simulink model "SPGF_FSK_0000_R2022b"  (R2022b)
settings: Solver=ode4  StartTime=0.0  StopTime=1.4  FixedStep=50e-6/50  RelTol=1e-3  EnableMultiTasking=on
undefined symbols (not defined in the file): D11, Delta
libraries: spsSeriesRLCBranchLib x1646, spsGroundLib x360, spsStairGeneratorLib x147, spsIdealSwitchLib x145, spsCurrentMeasurementLib x145, spsUniversalBridgeLib x76, spsThreePhaseSeriesRLCLoadLib x57, simulink x45, spsBistableLib x36, spsSequenceAnalyzerLib x31, spsThreePhaseParallelRLCLoadLib x20, spsThreePhaseTransformerTwoWindingsLib x20
(part 17 of 40)

== system SPGF_FSK_0000_R2022b/W12/concentrated ==
  Ccs/1 : spsSeriesRLCBranchLib/Series RLC Branch  LConnTagsString=__new0  RConnTagsString=__new0  BranchType=C  Resistance=190  Inductance=1e-3  SetiL0=off  InitialCurrent=0  Capacitance=-C_matrix(1,2)/2  Setx0=off  InitialVoltage=0  Measurements=None
  Ccs/2 : spsSeriesRLCBranchLib/Series RLC Branch  LConnTagsString=__new0  RConnTagsString=__new0  BranchType=C  Resistance=190  Inductance=1e-3  SetiL0=off  InitialCurrent=0  Capacitance=-C_matrix(1,2)/2  Setx0=off  InitialVoltage=0  Measurements=None
  Ccs2/1 : spsSeriesRLCBranchLib/Series RLC Branch  LConnTagsString=__new0  RConnTagsString=__new0  BranchType=C  Resistance=190  Inductance=1e-3  SetiL0=off  InitialCurrent=0  Capacitance=-C_matrix(3,4)/2  Setx0=off  InitialVoltage=0  Measurements=None
  Ccs2/2 : spsSeriesRLCBranchLib/Series RLC Branch  LConnTagsString=__new0  RConnTagsString=__new0  BranchType=C  Resistance=190  Inductance=1e-3  SetiL0=off  InitialCurrent=0  Capacitance=-C_matrix(3,4)/2  Setx0=off  InitialVoltage=0  Measurements=None
  Ccs2/3 : spsSeriesRLCBranchLib/Series RLC Branch  LConnTagsString=__new0  RConnTagsString=__new0  BranchType=R  Resistance=-Rg_matrix(3,4)*2  Inductance=1e-3  SetiL0=off  InitialCurrent=0  Capacitance=Rg_matrix(3,4)*2  Setx0=off  InitialVoltage=0  Measurements=None
  Ccs2/4 : spsSeriesRLCBranchLib/Series RLC Branch  LConnTagsString=__new0  RConnTagsString=__new0  BranchType=R  Resistance=-Rg_matrix(3,4)*2  Inductance=1e-3  SetiL0=off  InitialCurrent=0  Capacitance=Rg_matrix(3,4)*2  Setx0=off  InitialVoltage=0  Measurements=None
  Ccs3/1 : spsSeriesRLCBranchLib/Series RLC Branch  LConnTagsString=__new0  RConnTagsString=__new0  BranchType=C  Resistance=190  Inductance=1e-3  SetiL0=off  InitialCurrent=0  Capacitance=-C_matrix(5,6)/2  Setx0=off  InitialVoltage=0  Measurements=None
  Ccs3/2 : spsSeriesRLCBranchLib/Series RLC Branch  LConnTagsString=__new0  RConnTagsString=__new0  BranchType=C  Resistance=190  Inductance=1e-3  SetiL0=off  InitialCurrent=0  Capacitance=-C_matrix(5,6)/2  Setx0=off  InitialVoltage=0  Measurements=None
  Ccs3/3 : spsSeriesRLCBranchLib/Series RLC Branch  LConnTagsString=__new0  RConnTagsString=__new0  BranchType=R  Resistance=-Rg_matrix(5,6)*2  Inductance=1e-3  SetiL0=off  InitialCurrent=0  Capacitance=-C_matrix(5,6)/2  Setx0=off  InitialVoltage=0  Measurements=None
  Ccs3/4 : spsSeriesRLCBranchLib/Series RLC Branch  LConnTagsString=__new0  RConnTagsString=__new0  BranchType=R  Resistance=-Rg_matrix(5,6)*2  Inductance=1e-3  SetiL0=off  InitialCurrent=0  Capacitance=-C_matrix(5,6)/2  Setx0=off  InitialVoltage=0  Measurements=None
  Csg/2 : spsSeriesRLCBranchLib/Series RLC Branch  LConnTagsString=__new0  RConnTagsString=__new0  BranchType=C  Resistance=190  Inductance=1e-3  SetiL0=off  InitialCurrent=0  Capacitance=( C_matrix(1,2) + C_matrix(2,2) )/2  Setx0=off  InitialVoltage=0  Measurements=None
  Csg1/1 : spsSeriesRLCBranchLib/Series RLC Branch  LConnTagsString=__new0  RConnTagsString=__new0  BranchType=C  Resistance=190  Inductance=1e-3  SetiL0=off  InitialCurrent=0  Capacitance=( C_matrix(1,2) + C_matrix(2,2) )/2  Setx0=off  InitialVoltage=0  Measurements=None
  Csg2/1 : spsSeriesRLCBranchLib/Series RLC Branch  LConnTagsString=__new0  RConnTagsString=__new0  BranchType=C  Resistance=190  Inductance=1e-3  SetiL0=off  InitialCurrent=0  Capacitance=( C_matrix(3,4) + C_matrix(4,4) )/2  Setx0=off  InitialVoltage=0  Measurements=None
  Csg2/2 : spsSeriesRLCBranchLib/Series RLC Branch  LConnTagsString=__new0  RConnTagsString=__new0  BranchType=C  Resistance=190  Inductance=1e-3  SetiL0=off  InitialCurrent=0  Capacitance=( C_matrix(3,4) + C_matrix(4,4) )/2  Setx0=off  InitialVoltage=0  Measurements=None
  Csg3/1 : spsSeriesRLCBranchLib/Series RLC Branch  LConnTagsString=__new0  RConnTagsString=__new0  BranchType=C  Resistance=190  Inductance=1e-3  SetiL0=off  InitialCurrent=0  Capacitance=( C_matrix(5,6) + C_matrix(6,6) ) /2  Setx0=off  InitialVoltage=0  Measurements=None
  Csg3/2 : spsSeriesRLCBranchLib/Series RLC Branch  LConnTagsString=__new0  RConnTagsString=__new0  BranchType=C  Resistance=190  Inductance=1e-3  SetiL0=off  InitialCurrent=0  Capacitance=( C_matrix(5,6) + C_matrix(6,6) ) /2  Setx0=off  InitialVoltage=0  Measurements=None
  Ground{1..4} (4 alike) : spsGroundLib/Ground  LConnTagsString=a
  RL : spsMutualInductanceLib/Mutual Inductance  LConnTagsString=a|b|c|L4|L5|L6  RConnTagsString=A|B|C|R4|R5|R6  TypeOfMutual=Generalized mutual inductance  NumberOfWindings=6  SelfImpedance1=[1.1 1.1e-03]  SelfImpedance2=[ 1.1 1.1e-03]  ThreeWindings=on  SelfImpedance3=[ 1.1 1.1e-03]  MutualImpedance=[1.0 1.0e-03]  InductanceMatrix=L_matrix  ResistanceMatrix=R_matrix  Measurements=None
      settings: LibrarySourceBlock=sps_lib/Passives/Mutual Inductance
  Rcs*2 : spsSeriesRLCBranchLib/Series RLC Branch  LConnTagsString=__new0  RConnTagsString=__new0  BranchType=R  Resistance=-Rg_matrix(1,2)*2  Inductance=1e-3  SetiL0=off  InitialCurrent=0  Capacitance=Rg_matrix(1,2)*2  Setx0=off  InitialVoltage=0  Measurements=None
  Rgcs1/1 : spsSeriesRLCBranchLib/Series RLC Branch  LConnTagsString=__new0  RConnTagsString=__new0  BranchType=R  Resistance=-Rg_matrix(1,2)*2  Inductance=1e-3  SetiL0=off  InitialCurrent=0  Capacitance=Rg_matrix(1,2)*2  Setx0=off  InitialVoltage=0  Measurements=None
  Rgsg1/1 : spsSeriesRLCBranchLib/Series RLC Branch  LConnTagsString=__new0  RConnTagsString=__new0  BranchType=R  Resistance=(Rg_matrix(4,4)+Rg_matrix(3,4))*2  Inductance=1e-3  SetiL0=off  InitialCurrent=0  Capacitance=Rg_matrix(1,2)*2  Setx0=off  InitialVoltage=0  Measurements=None
  Rgsg1/2 : spsSeriesRLCBranchLib/Series RLC Branch  LConnTagsString=__new0  RConnTagsString=__new0  BranchType=R  Resistance=(Rg_matrix(2,2)+Rg_matrix(1,2))*2  Inductance=1e-3  SetiL0=off  InitialCurrent=0  Capacitance=Rg_matrix(1,2)*2  Setx0=off  InitialVoltage=0  Measurements=None
  Rgsg1/3 : spsSeriesRLCBranchLib/Series RLC Branch  LConnTagsString=__new0  RConnTagsString=__new0  BranchType=R  Resistance=(Rg_matrix(4,4)+Rg_matrix(3,4))*2  Inductance=1e-3  SetiL0=off  InitialCurrent=0  Capacitance=Rg_matrix(1,2)*2  Setx0=off  InitialVoltage=0  Measurements=None
  Rgsg1/4 : spsSeriesRLCBranchLib/Series RLC Branch  LConnTagsString=__new0  RConnTagsString=__new0  BranchType=R  Resistance=(Rg_matrix(2,2)+Rg_matrix(1,2))*2  Inductance=1e-3  SetiL0=off  InitialCurrent=0  Capacitance=Rg_matrix(1,2)*2  Setx0=off  InitialVoltage=0  Measurements=None
  Rsg*2 : spsSeriesRLCBranchLib/Series RLC Branch  LConnTagsString=__new0  RConnTagsString=__new0  BranchType=R  Resistance=(Rg_matrix(6,6)+Rg_matrix(5,6))*2  Inductance=1e-3  SetiL0=off  InitialCurrent=0  Capacitance=Rg_matrix(1,2)*2  Setx0=off  InitialVoltage=0  Measurements=None
  Rsg1/1 : spsSeriesRLCBranchLib/Series RLC Branch  LConnTagsString=__new0  RConnTagsString=__new0  BranchType=R  Resistance=(Rg_matrix(6,6)+Rg_matrix(5,6))*2  Inductance=1e-3  SetiL0=off  InitialCurrent=0  Capacitance=Rg_matrix(1,2)*2  Setx0=off  InitialVoltage=0  Measurements=None
  A : PMIOPort  Side=Left
  B : PMIOPort  Port=2  Side=Left
  C : PMIOPort  Port=3  Side=Left
  a : PMIOPort  Port=4  Side=Right
  b : PMIOPort  Port=5  Side=Right
  c : PMIOPort  Port=6  Side=Right
  connections:
  RL/LConn6 -- Ground3/LConn1 -- Rgsg1/2/LConn1 -- Csg/2/LConn1 -- Rcs*2/LConn1 -- Ccs/2/LConn1 -- RL/LConn2 -- RL/LConn4 -- Rgsg1/1/LConn1 -- Csg2/2/LConn1 -- Ccs2/3/LConn1 -- Ccs2/2/LConn1 -- Rsg*2/LConn1 -- Csg3/2/LConn1 -- Ccs3/3/LConn1 -- Ccs3/2/LConn1
  Rsg1/1/RConn1 -- Rgsg1/3/RConn1 -- Rgsg1/4/RConn1 -- Csg3/1/RConn1 -- Csg2/1/RConn1 -- Ground2/LConn1 -- Csg1/1/RConn1
  Rgsg1/3/LConn1 -- Ccs2/4/LConn1 -- Csg2/1/LConn1 -- Ccs2/1/LConn1 -- RL/RConn4 -- Rgsg1/4/LConn1 -- Rgcs1/1/LConn1 -- Csg1/1/LConn1 -- Ccs/1/LConn1 -- RL/RConn2 -- Ground4/LConn1 -- RL/RConn6 -- Ccs3/1/LConn1 -- Rsg1/1/LConn1 -- Ccs3/4/LConn1 -- Csg3/1/LConn1
  Rsg*2/RConn1 -- Rgsg1/1/RConn1 -- Rgsg1/2/RConn1 -- Csg3/2/RConn1 -- Csg2/2/RConn1 -- Ground1/LConn1 -- Csg/2/RConn1
  a/RConn1 -- RL/RConn1 -- Rgcs1/1/RConn1 -- Ccs/1/RConn1
  b/RConn1 -- RL/RConn3 -- Ccs2/4/RConn1 -- Ccs2/1/RConn1
  Ccs3/1/RConn1 -- c/RConn1 -- RL/RConn5 -- Ccs3/4/RConn1
  RL/LConn1 -- A/RConn1 -- Rcs*2/RConn1 -- Ccs/2/RConn1
  RL/LConn3 -- B/RConn1 -- Ccs2/3/RConn1 -- Ccs2/2/RConn1
  Ccs3/2/RConn1 -- C/RConn1 -- RL/LConn5 -- Ccs3/3/RConn1
